simulink library "MoonEphemeris_MathWorks"  (R2014b)
settings: Solver=ode45  StartTime=0.0  StopTime=10.0  RelTol=1e-3
settings Model: Creator=Hp  LastModifiedBy=Hp

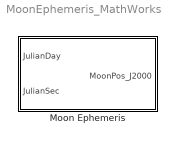
== system MoonEphemeris_MathWorks ==
  Moon Ephemeris : Subsystem

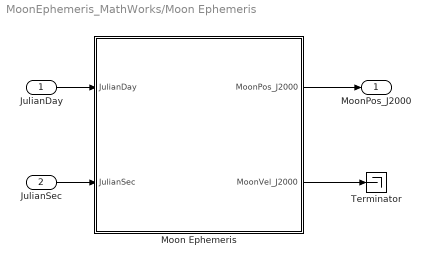
== system MoonEphemeris_MathWorks/Moon Ephemeris ==
  JulianDay : Inport
  JulianSec : Inport  Port=2
  Moon Ephemeris : MATLAB Function  TreatAsAtomicUnit=on
  Terminator : Terminator
  MoonPos_J2000 : Outport
  wires:
  JulianSec/1 -> Moon Ephemeris/2(JulianSec)
  JulianDay/1 -> Moon Ephemeris/1(JulianDay)
  Moon Ephemeris/1(MoonPos_J2000) -> MoonPos_J2000/1
  Moon Ephemeris/2(MoonVel_J2000) -> Terminator/1

== matlab function MoonEphemeris_MathWorks/Moon Ephemeris/Moon Ephemeris ==
  data: JulianDay input; MoonPos_J2000 output; JulianSec input; MoonVel_J2000 output
%**************************************************************************
%
%  A simple analytical lunar ephemeris model. Returns Lunar cartesian
%  coordinates (mean equator and equinox of epoch J2000).
%
% Input:
%  mjd        Modified Julian date
%
% Outputs:
%  r_moon    Moon position (m)
%  v_moon    Moon velocity (m/s)
%
%  Reference:
%    "An alternative lunar ephemeris model for on-board flight software use",
%    D. G. Simpson, Proceedings of the 1999 NASA/GSFC Flight Mechanics Symposium,
%    p. 175-184).
%
%  T = (JD - 2451545)/36525
%  X =  383.0e3 * SIN( 8399.685 * T + 5.381)
%      + 31.5e3 * SIN(   70.990 * T + 6.169)
%      + 10.6e3 * SIN(16728.377 * T + 1.453)
%      +  6.2e3 * SIN( 1185.622 * T + 0.481)
%      +  3.2e3 * SIN( 7143.070 * T + 5.017)
%      +  2.3e3 * SIN(15613.745 * T + 0.857)
%      +  0.8e3 * SIN( 8467.263 * T + 1.010)
%  Y =  351.0e3 * SIN( 8399.687 * T + 3.811)
%      + 28.9e3 * SIN(   70.997 * T + 4.596)
%      + 13.7e3 * SIN( 8433.466 * T + 4.766)
%      +  9.7e3 * SIN(16728.380 * T + 6.165)
%      +  5.7e3 * SIN( 1185.667 * T + 5.164)
%      +  2.9e3 * SIN( 7143.058 * T + 0.300)
%      +  2.1e3 * SIN(15613.755 * T + 5.565)
%  Z =  153.2e3 * SIN( 8399.672 * T + 3.807)
%      + 31.5e3 * SIN( 8433.464 * T + 1.629)
%      + 12.5e3 * SIN(   70.996 * T + 4.595)
%      +  4.2e3 * SIN(16728.364 * T + 6.162)
%      +  2.5e3 * SIN( 1185.645 * T + 5.167)
%      +  3.0e3 * SIN(  104.881 * T + 2.555)
%      +  1.8e3 * SIN( 8399.116 * T + 6.248)
%
%**************************************************************************
function [MoonPos_J2000, MoonVel_J2000] = MoonEphem(JulianDay, JulianSec)

century2day = 36525;
day2sec = 86400;

xcoeffs = [383.0e3, 31.5e3, 10.6e3, 6.2e3, 3.2e3, 2.3e3, 0.8e3];
ycoeffs = [351.0e3, 28.9e3, 13.7e3, 9.7e3, 5.7e3, 2.9e3, 2.1e3];
zcoeffs = [153.2e3, 31.5e3, 12.5e3, 4.2e3, 2.5e3, 3.0e3, 1.8e3];
xa = [8399.685, 70.990, 16728.377, 1185.622, 7143.070, 15613.745, 8467.263];
xp = [5.381, 6.169, 1.453, 0.481, 5.017, 0.857, 1.010];
ya = [8399.687, 70.997, 8433.466, 16728.380, 1185.667, 7143.058, 15613.755];
yp = [3.811, 4.596, 4.766, 6.165, 5.164, 0.300, 5.565];
za = [8399.672, 8433.464, 70.996, 16728.364, 1185.645, 104.881, 8399.116];
zp = [3.807, 1.629, 4.595, 6.162, 5.167, 2.555, 6.248];
vxcoeffs = xcoeffs.*xa;
vycoeffs = ycoeffs.*ya;
vzcoeffs = zcoeffs.*za;

mjd = JulianDay+JulianSec/86400+51544; % Modified JulianDay 

t = (mjd - 51544.5)/century2day; % time in Julian centuries from J2000

xterms = xa * t + xp;
yterms = ya * t + yp;
zterms = za * t + zp;

MoonPos_J2000 = zeros(3,1);

MoonPos_J2000(1) = 1e3*dot(xcoeffs, sin(xterms));
MoonPos_J2000(2) = 1e3*dot(ycoeffs, sin(yterms));
MoonPos_J2000(3) = 1e3*dot(zcoeffs, sin(zterms));

MoonVel_J2000 = zeros(3,1);
% v_moon is just d(r_moon)/dt
MoonVel_J2000(1) =  1e3*dot(vxcoeffs, cos(xterms))/(century2day * day2sec);
MoonVel_J2000(2) =  1e3*dot(vycoeffs, cos(yterms))/(century2day * day2sec);
MoonVel_J2000(3) =  1e3*dot(vzcoeffs, cos(zterms))/(century2day * day2sec);

end
